simulink model "Viterbi_Simulink_Model"  (R2025b)
settings: Solver=FixedStepDiscrete  StartTime=0.0  StopTime=1e5  FixedStep=1  RelTol=1e-3
values from neighbouring files (symbols this model uses):
  CODE_RATE = 1/2    (= 0.5)    [cosim_rtl_ber_sweep.m]
  EbN0_dB = p.Results.EbN0(:).'    [cosim_rtl_ber_sweep.m]
undefined symbols (not defined in the file or in its folder): SOFT_BITS
libraries: commcnvcod2 x3, commsink2 x2, commdigbbndpm3 x2, commchan3 x1, commrandsrc3 x1, commsrccod2 x1
settings Model: Creator=andre  LastModifiedBy=andre

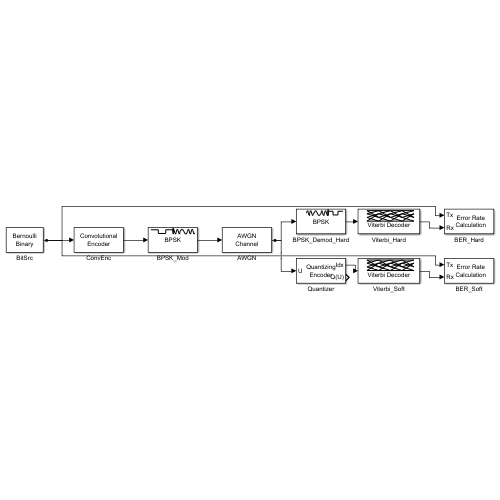
[thumbnail: Simulink's stored preview of the top-level diagram]
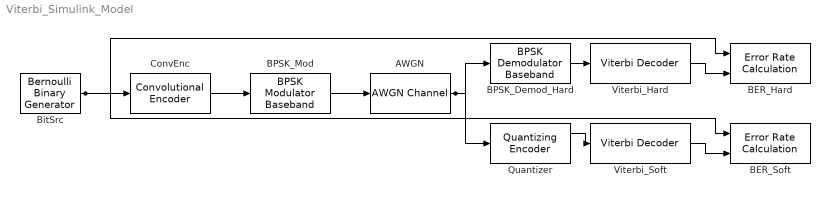
== system Viterbi_Simulink_Model ==
  AWGN : commchan3/AWGN Channel  LegacyMode=off  NoiseMethod="Signal to noise ratio  (SNR)"  noiseMode="Signal to noise ratio  (SNR)"  EbNo=10  EsNo=10  SNR=10  BitsPerSymbol=1  SignalPower=1  SpecifySymbolPeriod=off  SamplesPerSymbol=1  SymbolPeriod=1  VarianceSource=Parameter  Variance=1/(2*CODE_RATE*10^(EbN0_dB/10))  RandomStream=Global stream  Seed=67  SimulateUsing=Code generation
  BER_Hard : commsink2/Error Rate Calculation  N=0  st_delay=0  cp_mode=Entire frame  subframe=[]  PMode=Workspace  WsName=BER_hard  RsMode2=off  stop=off  numErr=100  maxBits=1e6
  BER_Soft : commsink2/Error Rate Calculation  N=0  st_delay=0  cp_mode=Entire frame  subframe=[]  PMode=Workspace  WsName=BER_soft  RsMode2=off  stop=off  numErr=100  maxBits=1e6
  BPSK_Demod_Hard : commdigbbndpm3/BPSK Demodulator Baseband  DecType=Hard decision  VarSource=Dialog  Variance=1  Ph=0  outDtype=Inherit via internal rule  derotateFactorWordLen=16  derotateFactorDataTypeStr=Inherit: Same word length as input  derotateFactorLastDataTypeStr=Inherit: Same word length as input
  BPSK_Mod : commdigbbndpm3/BPSK Modulator Baseband  Ph=0  outDtype=double  outWordLen=16  outUDDataType=sfix(16)  outFracLenMode=Best precision  outFracLen=15  outDataTypeStr=double  outLastDataTypeStr=double
  BitSrc : commrandsrc3/Bernoulli Binary Generator  ProbabilityOfZero=0.5  SeedSource=Auto  Seed=0  SampleTime=1  SamplesPerFrame=1  OutputDataType=double  SimulateUsing=Interpreted execution
  ConvEnc : commcnvcod2/Convolutional Encoder  trellis=TRELLIS  opMode=Continuous  DelayedResetAction=off  hasIniStPort=off  hasFinStPort=off  usePuncVector=off  punctureVector=[1; 1; 0; 1; 0; 1]  reset=Unused parameter value
  Quantizer : commsrccod2/Quantizing Encoder  partition=linspace(-1, 1, 2^SOFT_BITS - 1)  codebook=0:(2^SOFT_BITS - 1)  idxDType=double
  Viterbi_Hard : commcnvcod2/Viterbi Decoder  trellis=TRELLIS  isPunctured=off  punctureVector=[1; 1; 0; 1; 0; 1]  erasures=off  dectype=Hard decision  nsdecb=4  runSigValErrCheck=off  tbdepth=TB_DEPTH  opmode=Truncated  reset=off  delayedResetAction=off  smWordLength=16  outDataType=Inherit via internal rule
  Viterbi_Soft : commcnvcod2/Viterbi Decoder  trellis=TRELLIS  isPunctured=off  punctureVector=[1; 1; 0; 1; 0; 1]  erasures=off  dectype=Soft decision  nsdecb=SOFT_BITS  runSigValErrCheck=off  tbdepth=TB_DEPTH  opmode=Truncated  reset=off  delayedResetAction=off  smWordLength=16  outDataType=Inherit via internal rule
  wires:
  BitSrc/1 -> ConvEnc/1, BER_Hard/1, BER_Soft/1
  ConvEnc/1 -> BPSK_Mod/1
  BPSK_Mod/1 -> AWGN/1
  AWGN/1 -> BPSK_Demod_Hard/1, Quantizer/1
  BPSK_Demod_Hard/1 -> Viterbi_Hard/1
  Viterbi_Hard/1 -> BER_Hard/2
  Quantizer/1 -> Viterbi_Soft/1
  Viterbi_Soft/1 -> BER_Soft/2
